simulink model "sdruFRSGMRSRx"  (R2014a)
settings: Solver=FixedStepDiscrete  SolverMode=SingleTasking  StartTime=0.0  StopTime=inf  RelTol=1e-3
PreLoadFcn:
  | FRSRxParams = getParamsSdruFRSGMRSRxDemo;
  | 
  | % The following parameters cannot be put into the FRSRxParams structure,
  | % because they are used as arguments in a MATLAB Function block.
  | frs_coeff = FRSRxParams.GoertzelCoefficients;
  | frs_Fs = FRSRxParams.SampleRate;
  | frs_toneFreqs = FRSRxParams.ToneFrequencies;
  | frs_decodeBlockSize = FRSRxParams.CTCSSDecodeBlockLength;
InitFcn:
  | FRSRxParams = getParamsSdruFRSGMRSRxDemo;
  | 
  | % The following parameters cannot be put into the FRSRxParams structure,
  | % because they are used as arguments in a MATLAB Function block.
  | frs_coeff = FRSRxParams.GoertzelCoefficients;
  | frs_Fs = FRSRxParams.SampleRate;
  | frs_toneFreqs = FRSRxParams.ToneFrequencies;
  | frs_decodeBlockSize = FRSRxParams.CTCSSDecodeBlockLength;
undefined symbols (not defined in the file or in its folder): a1, b0, b1, dfilt, fdesignblkfcn, gcbh, mfilt
libraries: dsparch4 x2, commrfcorlib x1, dspmlti4 x1, dspsigops x1, dspsnks4 x1, sdrublksprivate x1, commsdrhw_v2 x1
CloseFcn:
  | clear FRSRxParams frs_Fs frs_channelFilt frs_toneFreqs frs_coeff frs_decodeBlockSize
Description:
  | This model uses Simulink(R) to receive a Family Radio Service (FRS) signal from Universal Software Radio Peripheral (USRP) hardware.
settings Model: Creator=The MathWorks Inc.
settings DataIOCC: LimitDataPoints=off  SignalLoggingSaveFormat=ModelDataLogs  SaveOutput=off  SignalLogging=off  DSMLogging=off  SaveTime=off
settings OptimizationCC: ExpressionDepthLimit=2147483647  SimCompilerOptimization=On
settings DebuggingCC: UnderspecifiedInitializationDetection=Classic  InheritedTsInSrcMsg=none  MultiTaskCondExecSysMsg=none  ParameterPrecisionLossMsg=none  FcnCallInpInsideContextMsg=UseLocalSettings  StateNameClashWarn=warning
settings HardwareCC: TargetBitPerLong=64  TargetBitPerPointer=64  TargetLongLongMode=on  TargetIntDivRoundTo=Zero  TargetEndianess=LittleEndian  TargetWordSize=64  TargetHWDeviceType=Generic->MATLAB Host Computer  ProdEqTarget=off
settings SFSimCC: SFSimEnableDebug=off  SFSimOverflowDetection=off  SimIntegrity=off
settings RTWCC: CustomSourceCode=|
  | #include <stdio.h>
  | #include <stdlib.h>
settings GRTTargetCC: CombineOutputUpdateFcns=off  GRTInterface=on

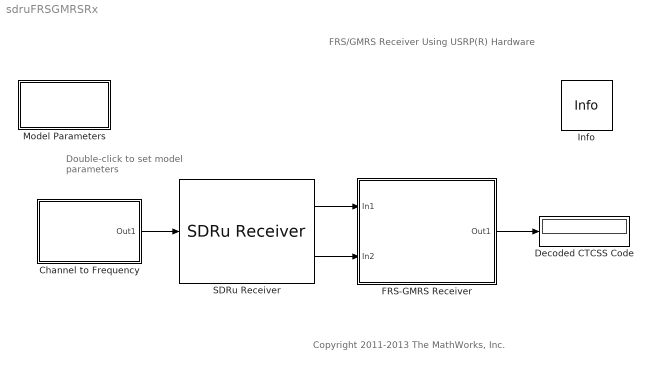
== system sdruFRSGMRSRx ==
  note: Copyright 2011-2013 The MathWorks, Inc.
  note: FRS/GMRS Receiver Using USRP(R) Hardware
  note: Double-click to
      | set model parameters
  Channel to Frequency : Subsystem
      mask Display: disp('Channel to\nFrequency');
  Decoded CTCSS Code : Display
  FRS-GMRS Receiver : Subsystem
      mask Display: disp('FRS-GMRS Receiver');
  Info : sdrublksprivate/Info  SystemSampleTime=-1
  Model Parameters : Subsystem  mask(Model Parameters){channel=12, code=5, decodeThresh=0.1}
      mask prompts: channel "Channel (1 to 14):"; code "CTCSS Code (0 to 38):"; decodeThresh "Average signal threshold for squelch:"
      mask help: Specifies model parameters for a simulation run.
      mask init:
      | usrpFRSGMRS_mask(gcbh, 'init', 'rec', channel, code, decodeThresh);
      mask Help: web(usrpdhelp, '-helpbrowser');
      mask Display: disp('Model\nParameters');
  SDRu Receiver : commsdrhw_v2/SDRu Receiver  rxtx=rx  USRP2_IP='192.168.10.2'  centerFrequency=2.45e9  centerFrequencySrc=Input port  loOffset=0  loOffsetSrc=Dialog  gain=0  gainSrc=Dialog  decimInterp=500  decimInterpSrc=Dialog  USRP2_IP_NUM=[49 57 50 46 49 54 56 46 49 48 46 50]  frameLength=4000  outputDatatype=single  overrunUnderrunPort=off  sampleTime=1/FRSRxParams.FrontEndSampleRate  HOST_DATA_PORT=30000  HOST_CONTROL_PORT=30002  USRP2_DATA_PORT=32769  USRP2_CONTROL_PORT=32768  bufferMode=Continuous streaming  EnableBurstMode=off  NumFramesInBurst=100
  wires:
  Channel to Frequency/1(Out1) -> SDRu Receiver/1
  FRS-GMRS Receiver/1(Out1) -> Decoded CTCSS Code/1
  SDRu Receiver/2 -> FRS-GMRS Receiver/2(In2)
  SDRu Receiver/1 -> FRS-GMRS Receiver/1(In1)

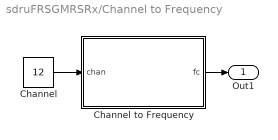
== system sdruFRSGMRSRx/Channel to Frequency ==
  Channel : Constant  Value=12  VectorParams1D=off  OutDataTypeStr=uint16  SampleTime=-1  FramePeriod=-1
  Channel to Frequency : MATLAB Function  TreatAsAtomicUnit=on
  Out1 : Outport
  wires:
  Channel/1 -> Channel to Frequency/1(chan)
  Channel to Frequency/1(fc) -> Out1/1

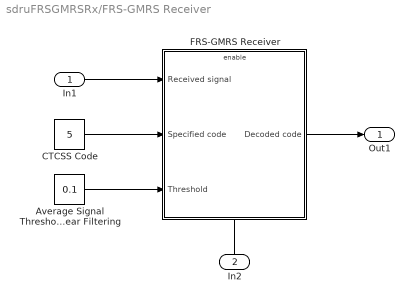
== system sdruFRSGMRSRx/FRS-GMRS Receiver ==
  In1 : Inport
  In2 : Inport  Port=2
  Average Signal Threshold for Nonlinear Filtering : Constant  Value=0.1  VectorParams1D=off  OutDataTypeStr=single  FramePeriod=-1
  CTCSS Code : Constant  Value=5  OutDataTypeStr=uint8
  FRS-GMRS Receiver : Subsystem  TreatAsAtomicUnit=on
  Out1 : Outport
  wires:
  CTCSS Code/1 -> FRS-GMRS Receiver/2(Specified code)
  Average Signal Threshold for Nonlinear Filtering/1 -> FRS-GMRS Receiver/3(Threshold)
  In1/1 -> FRS-GMRS Receiver/1(Received signal)
  FRS-GMRS Receiver/1(Decoded code) -> Out1/1
  In2/1 -> FRS-GMRS Receiver/Enable

== system sdruFRSGMRSRx/Model Parameters ==
  note: This subsystem is empty.
      | It is used for setting parameter values (in the mask).

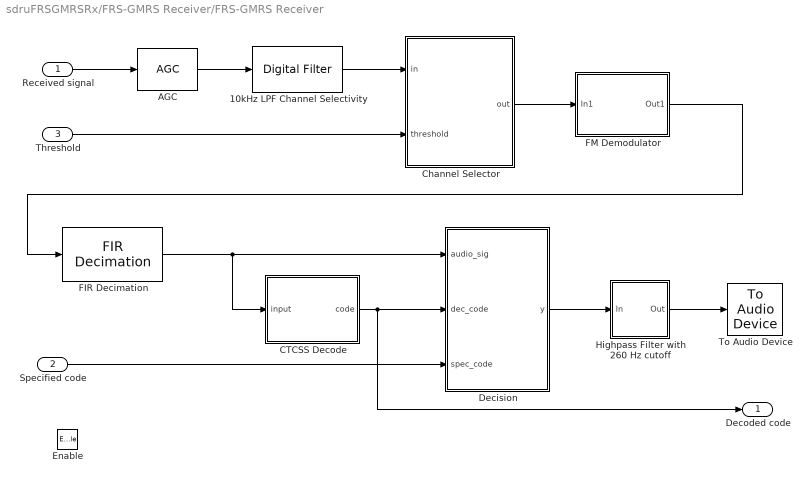
== system sdruFRSGMRSRx/FRS-GMRS Receiver/FRS-GMRS Receiver ==
  Received signal : Inport
  Specified code : Inport  Port=2
  Threshold : Inport  Port=3
  Enable : EnablePort
  10kHz LPF Channel Selectivity : dsparch4/Digital Filter  TypePopup=IIR (poles & zeros)  IIRFiltStruct=Biquad direct form I transposed (SOS)  AllPoleFiltStruct=Direct form  FIRFiltStruct=Direct form  CoeffSource=Specify via dialog  NumCoeffs=[b0 b1]  DenCoeffs=[1 a1]  BiQuadCoeffs=FMMono.Deemp5_Mono_sos  LatticeCoeffs=[0.2 0.4]  denIgnore=on  FiltPerSampPopup=One filter per frame  IC=0  ICnum=0  ICden=0  roundingMode=Floor  overflowMode=off  ScaleValues=FMMono.Deemp5_Mono_SV  scaleValueFracLength=14  stageInFracLength=15  stageOutFracLength=15  FilterSource=dfilt object  dfiltObjectName=frs_channelFilt  InputProcessing=Columns as channels (frame based)
  AGC : commrfcorlib/AGC  SimulateUsing=Code generation  DetectorMethod=Rectifier  LoopMethod=Linear  UpdatePeriod=1  StepSize=1  MaximumGain=1e6  GainOutputPort=off
  CTCSS Decode : MATLAB Function  TreatAsAtomicUnit=on
  Channel Selector : MATLAB Function  TreatAsAtomicUnit=on
  Decision : MATLAB Function  TreatAsAtomicUnit=on
  FIR Decimation : dspmlti4/FIR Decimation  h=fir1(35,0.4)  D=2  filtStruct=Direct form  framing=Enforce single-rate processing  inputOffset=0  outputBufInitCond=0  InputProcessing=Columns as channels (frame based)  firstCoeffDataTypeStr=Inherit: Same word length as input  firstCoeffLastDataTypeStr=Inherit: Same word length as input  firstCoeffMin=[]  firstCoeffMax=[]  outputDataTypeStr=Inherit: Same as accumulator  outputLastDataTypeStr=Inherit: Same as accumulator  outputMin=[]  outputMax=[]  roundingMode=Floor  overflowMode=off  FilterSource=Filter object  FilterObject=mfilt.firdecim(25)
      settings: allowOverrides=off
  FM Demodulator : Subsystem
  Highpass Filter with 260 Hz cutoff : Subsystem  DialogController=fdesignblkfcn  InitFcn=fdesignblkfcn(gcbh, {'InitFcn'});  mask(Highpass Filter){}
      mask help: Design a highpass filter
      settings: CopyFcn=fdesignblkfcn(gcbh, {'CopyFcn'});
      mask Help: helpview(mapfilelocation('dsp'), 'dsphighpassfilter');
      mask Display: disp('Highpass')
  To Audio Device : dspsnks4/To Audio Device  deviceName=Default  inheritSampleRate=on  sampleRate=7812  deviceDatatype=Determine from input data type  autoBufferSize=on  bufferSize=4096  queueDuration=1.0  defaultOutputChannelMapping=on  outputChannelMapping=1
  Decoded code : Outport
  wires:
  Received signal/1 -> AGC/1
  FM Demodulator/1(Out1) -> FIR Decimation/1
  Channel Selector/1(out) -> FM Demodulator/1(In1)
  10kHz LPF Channel Selectivity/1 -> Channel Selector/1(in)
  AGC/1 -> 10kHz LPF Channel Selectivity/1
  Decision/1(y) -> Highpass Filter with 260 Hz cutoff/1(In)
  FIR Decimation/1 -> Decision/1(audio_sig), CTCSS Decode/1(input)
  Highpass Filter with 260 Hz cutoff/1(Out) -> To Audio Device/1
  Specified code/1 -> Decision/3(spec_code)
  Threshold/1 -> Channel Selector/2(threshold)
  CTCSS Decode/1(code) -> Decoded code/1, Decision/2(dec_code)

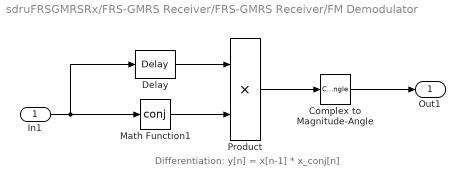
== system sdruFRSGMRSRx/FRS-GMRS Receiver/FRS-GMRS Receiver/FM Demodulator ==
  note: Differentiation:
      | y[n] = x[n-1] * x_conj[n]
  In1 : Inport
  Complex to Magnitude-Angle : ComplexToMagnitudeAngle  Output=Angle
  Delay : dspsigops/Delay  InputProcessing=Columns as channels (frame based)  dly_unit=Samples  delay=1  ic_detail=off  dif_ic_for_ch=off  dif_ic_for_dly=off  ic=0  reset_popup=None
  Math Function1 : Math  Operator=conj  SaturateOnIntegerOverflow=on
  Product : Product  RndMeth=Zero
  Out1 : Outport
  wires:
  Product/1 -> Complex to Magnitude-Angle/1
  Delay/1 -> Product/1
  In1/1 -> Delay/1, Math Function1/1
  Math Function1/1 -> Product/2
  Complex to Magnitude-Angle/1 -> Out1/1

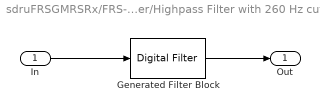
== system sdruFRSGMRSRx/FRS-GMRS Receiver/FRS-GMRS Receiver/Highpass Filter with 260 Hz cutoff ==
  In : Inport
  Generated Filter Block : dsparch4/Digital Filter  Tag=BlockMethodSubSystem  TypePopup=FIR (all zeros)  IIRFiltStruct=Direct form II transposed  AllPoleFiltStruct=Direct form  FIRFiltStruct=Direct form  CoeffSource=Specify via dialog  NumCoeffs=[-6.70616028565453e-05 0.0231597313321167 -0.00195810845100935 -0.00212362980418861 -0.00230222773581397 -0.0025599768128842 -0.00282265928211798 -0.00307311599192571 -0.00326318669112262 -0.00335250278736369 -0.00331109256996352 -0.00311389345721505 -0.00274282611939017 -0.00220068794468058 -0.00149387320797647 -0.000649320354931734 0.000297110329982477 0.00129670303353386 0.00229428253834002 0.00322554840796166 0.00403000858179781 0.00464393327285169 0.00501542768358974 0.00509972777786509 0.00486965035921977 0.00431249559013671 0.00343906740514331 0.00227631462301952 0.000876326047773495 -0.00069412704606117 -0.00234850149834989 -0.00399137185354097 -0.00551672234003995 -0.00682106998144928 -0.00780166305052705 -0.00837130525938158 -0.00845674938124254 -0.00801137025801248 -0.00701341567888291 -0.0054761667431134 -0.00344240536182248 -0.000992626425614734 0.00176443098873577 0.00468850257800923 0.00761872043044714 0.0103751740337081 0.0127730216412211 0.0146241855902817 0.0157548354225377 0.0160076397392388 0.0152557037804291 0.0134077817816603 0.0104168060444964 0.0062808572184121 0.00105216341319874 -0.00517073370997429 -0.0122394968364422 -0.0199603705716491 -0.0281082943720028 -0.0364254857446745 -0.0446379950846675 -0.0524700022388859 -0.0596483625379307 -0.0659079289391955 -0.0710550090012872 -0.0748498268583931 -0.0771906571007537 0.921948829829737 -0.0771906571007537 -0.0748498268583931 -0.0710550090012872 -0.0659079289391955 -0.0596483625379307 -0.0524700022388859 -0.0446379950846675 -0.0364254857446745 -0.0281082943720028 -0.0199603705716491 -0.0122394968364422 -0.00517073370997429 0.00105216341319874 0.0062808572184121 0.0104168060444964 0.0134077817816603 0.0152557037804291 0.0160076397392388 0.0157548354225377 0.0146241855902817 0.0127730216412211 0.0103751740337081 0.00761872043044714 0.00468850257800923 0.00176443098873577 -0.000992626425614734 -0.00344240536182248 -0.0054761667431134 -0.00701341567888291 -0.00801137025801248 -0.00845674938124254 -0.00837130525938158 -0.00780166305052705 -0.00682106998144928 -0.00551672234003995 -0.00399137185354097 -0.00234850149834989 -0.00069412704606117 0.000876326047773495 0.00227631462301952 0.00343906740514331 0.00431249559013671 0.00486965035921977 0.00509972777786509 0.00501542768358974 0.00464393327285169 0.00403000858179781 0.00322554840796166 0.00229428253834002 0.00129670303353386 0.000297110329982477 -0.000649320354931734 -0.00149387320797647 -0.00220068794468058 -0.00274282611939017 -0.00311389345721505 -0.00331109256996352 -0.00335250278736369 -0.00326318669112262 -0.00307311599192571 -0.00282265928211798 -0.0025599768128842 -0.00230222773581397 -0.00212362980418861 -0.00195810845100935 0.0231597313321167 -6.70616028565453e-05]  DenCoeffs=[1 0.1]  BiQuadCoeffs=[1 0.3 0.4 1 0.1 0.2]  LatticeCoeffs=[0.2 0.4]  denIgnore=on  FiltPerSampPopup=One filter per frame  IC=0  ICnum=0  ICden=0  roundingMode=Floor  overflowMode=off  ScaleValues=1  scaleValueFracLength=14  stageInFracLength=15  stageOutFracLength=15  FilterSource=Specify via dialog  dfiltObjectName=dfilt.dffir([1 2 1])  InputProcessing=Columns as channels (frame based)
  Out : Outport
  wires:
  Generated Filter Block/1 -> Out/1
  In/1 -> Generated Filter Block/1

== matlab function sdruFRSGMRSRx/FRS-GMRS Receiver/FRS-GMRS Receiver/CTCSS Decode ==
  data: input input; code output int8; frs_toneFreqs parameter; frs_coeff parameter; frs_decodeBlockSize parameter
function code  = CTCSS_Decode(input, frs_toneFreqs, frs_coeff, frs_decodeBlockSize)
%#codegen
% CTCSS decoder for use in a tone squelch system.
%
% Requires identification of one of a set of tones in the audio stream.
% Input is a frame of audio samples at a sample rate of (close to) 8kHz.
%
% Each time the function is called when a frame of samples comes in. It
% changes the state of the function, s(n), s(n-1), s(n-2). When a block of
% samples passes through (block size specified by frs_decodeBlockSize ),
% the power at each frequency is computed by Goertzel algorithm and the
% state is cleared to zero, preparing for the next block. The block size
% could be much larger than the frame size. 
%
% Below is the frequency table for private codes. 
% 
% PL   Hz     PL   Hz      PL   Hz
% --  ----    --  -----    --  -----
%  1  67.0    12  100.0    32  203.5
%  2  71.9    13  103.5    33  210.7
%  3  74.4    14  107.2    34  218.1
%  4  77.0    15  110.9    35  225.7
%  5  79.7    16  114.8    36  233.6
%  6  82.5    17  118.8    37  241.8
%  7  85.4    18  123.0    38  250.3
%  8  88.5    19  127.3
%  9  91.5    20  131.8
% 10  94.8    21  136.5
% 11  97.4    22  141.3
%             23  146.2
%             24  151.4
%             25  156.7
%             26  162.2
%             27  167.9
%             28  173.8
%             29  179.9
%             30  186.2
%             31  192.8

nTones = length(frs_toneFreqs);

persistent  s_d1 s_d2 s maxPowerIdx nProcessed

if isempty(s_d1)
    s_d1 = coder.nullcopy(single(zeros(nTones,1)));% s_d1 = s(n-1)
    s_d2 = coder.nullcopy(single(zeros(nTones,1)));% s_d2 = s(n-2)
    s = coder.nullcopy(single(zeros(nTones,1))); % s = s(n)
    nProcessed = 0;
    maxPowerIdx = 0; 
end

frameSize = length(input);

% The number of sample needs to be processed
nSampleProc = min(frameSize, frs_decodeBlockSize - nProcessed);

for i = 1:nSampleProc
	inputVec = repmat(input(i), nTones,1);
	s  = inputVec + frs_coeff .* s_d1 - s_d2; % s(n) = x(n) + 2cos(2*pi*w)s(n-1) - s(n-2)
	s_d2 = s_d1;
	s_d1 = s;
end

nProcessed  = nProcessed + nSampleProc;

% if a block is done
if (nProcessed == frs_decodeBlockSize)
	
	power = s_d2.^2 + s_d1.^2 - frs_coeff .* s_d2 .* s_d1;

    if (any(power ~= 0))
        [~, maxPowerIdx] = max(power);
    end

    % clear the state
	s_d1 = single(zeros(nTones,1));
	s_d2 = single(zeros(nTones,1));
	
    % next block starts, process the remaining samples in the current frame
	for i = nSampleProc + 1 : frameSize
		inputVec = repmat(input(i), nTones,1);
		s  = inputVec + frs_coeff .* s_d1 - s_d2;
		s_d2 = s_d1;
		s_d1 = s;
	end
	nProcessed = frameSize - nSampleProc;

end

code = int8(maxPowerIdx);

== matlab function sdruFRSGMRSRx/Channel to Frequency/Channel to Frequency ==
  data: chan input uint16; fc output double
function fc = ChanToFreq(chan)
%#codegen
% Map integer channel number to FRS/GMRS center frequencies

fc = convertChan2FreqFRSGMRSDemo(chan);

== matlab function sdruFRSGMRSRx/FRS-GMRS Receiver/FRS-GMRS Receiver/Decision ==
  data: audio_sig input; dec_code input; y output; spec_code input
function y  = decision(audio_sig, dec_code, spec_code)
%#codegen

% If the decoded code equals to pre-specified code, or the pre-specified
% code is 0 (no CTCSS), the audio signal goes through, otherwise, output
% zero.

if ((dec_code == spec_code) || (spec_code == 0))
    y = audio_sig;
else
    y = single(zeros(length(audio_sig),1));
end

== matlab function sdruFRSGMRSRx/FRS-GMRS Receiver/FRS-GMRS Receiver/Channel Selector ==
  data: in input; out output; threshold input
function out = channelSelector(in, threshold)
%#codegen
% Compute the average power of the input signal, if
% it is greater than a threshold, let the signal go through, otherwise,
% mute. 

len = length(in); 
power = sum(abs(in)) / len;

if (power >= threshold)
    out = in;
else 
    out = single(zeros(len,1));
end
